simulink model "satellite"  (R2025b)
settings: Solver=ode4  StartTime=0.0  StopTime=100  FixedStep=0.001  RelTol=1e-3
values from neighbouring files (symbols this model uses):
  A_mw = [ ... (first row only)    [init_params.m]
  A_w = [ ... (first row only)    [init_params.m]
  angle0 = eAR'    [init_params.m]
  area_d = 4    [init_params.m]
  area_s = 2    [init_params.m]
  B_mw = [ ... (first row only)    [init_params.m]
  C_bus = 0.001    [init_params.m]
  C_mw = [ ... (first row only)    [init_params.m]
  Cd = 2.2    [init_params.m]
  cos_g_max = cos(gamma_max)    [init_params.m]
  Cr = 1.2    [init_params.m]
  D_max = 0.95    [init_params.m]
  D_min = V_bus_ref / V_oc    (= 0.677637947725)    [init_params.m]
  Delta_D = 0.001    [init_params.m]
  dP_th = 0.05    [init_params.m]
  eta = 0.7    [init_params.m]
  eta_buck = 0.9    [init_params.m]
  eta_chg = 0.95    [init_params.m]
  f = 2.2e9    (= 2200000000)    [init_params.m]
  Gr_dB = 20    [init_params.m]
  Gt_dB = 3    [init_params.m]
  H = 50e3    (= 50000)    [init_params.m]
  h_ref = 400e3    (= 400000)    [init_params.m]
  hat_s = [1;0;0]    [init_params.m]
  I_chg_max = 8    [init_params.m]
  I_dis_max = 10    [init_params.m]
  I_sc = 10.38    [init_params.m]
  Iw = 0.02    [init_params.m]
  J2 = 1.08262668e-3    (= 0.00108262668)    [init_params.m]
  Jx = 10    [init_params.m]
  Jy = 12    [init_params.m]
  Jz = 8    [init_params.m]
  K_w = -A_w' * inv(A_w * A_w')    [init_params.m]
  Kd = [ ... (first row only)    [init_params.m]
  Kp = [ ... (first row only)    [init_params.m]
  m = 500    [init_params.m]
  mu = 3.986004418e14    (= 398600441800000)    [init_params.m]
  n_solar = [1;0;0]    [init_params.m]
  omegaE = 7.2921159e-5    (= 7.2921159e-05)    [init_params.m]
  P0 = 4.56e-6    (= 4.56e-06)    [init_params.m]
  P_adcs = 20    [init_params.m]
  P_base = 50    [init_params.m]
  P_cc = 220/V_bus_ref    (= 7.85714285714)    [init_params.m]
  P_comm = 40    [init_params.m]
  P_trickle = 14/V_bus_ref    (= 0.5)    [init_params.m]
  Pt_dBW = 10    [init_params.m]
  Q = 20    [init_params.m]
  Q0 = [0.6;0.8;0;0]    [init_params.m]
  Rb = 0.2    [init_params.m]
  Re = 6378137    [init_params.m]
  rho_ref = 3e-12    [init_params.m]
  SOC0 = 0.6    [init_params.m]
  SOC1 = 0.2    [init_params.m]
  SOC2 = 0.8    [init_params.m]
  SOC_low_adcs = 0.1    [init_params.m]
  SOC_low_comm = 0.2    [init_params.m]
  sta_vec = Re * [ ... (first row only)    [init_params.m]
  T_max = 0.05    [init_params.m]
  V_bus_ref = 28    [init_params.m]
  V_max = 33    [init_params.m]
  V_min = 24    [init_params.m]
  V_oc = 41.32    [init_params.m]
  vx0 = 0    [init_params.m]
  vy0 = 7546    [init_params.m]
  vz0 = 0    [init_params.m]
  w0 = [0;0;0]    [init_params.m]
  x0 = 7e6    (= 7000000)    [init_params.m]
  y0 = 0    [init_params.m]
  z0 = 0    [init_params.m]
libraries: matrix_library x8
settings Model: PauseTimes=900  Creator=NUAA  LastModifiedBy=NUAA

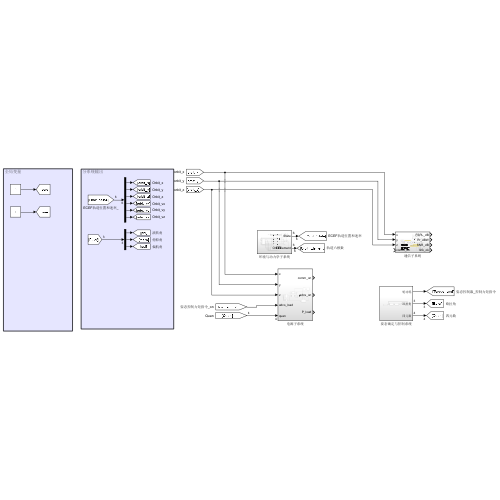
[thumbnail: Simulink's stored preview of the top-level diagram]
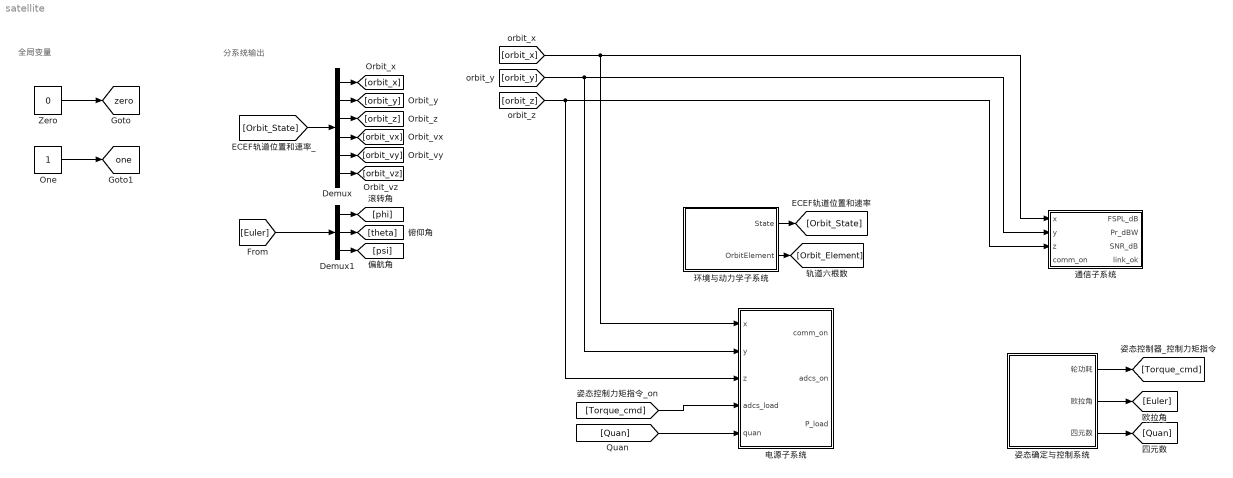
== system satellite ==
  note: 全局变量
  note: 分系统输出
  Demux : Demux  Outputs=6
  Demux1 : Demux  Outputs=3
  One : Constant  OutDataTypeStr=Inherit: Inherit via back propagation
  Zero : Constant  Value=0  OutDataTypeStr=Inherit: Inherit via back propagation
  姿态确定与控制系统 : Subsystem
  环境与动力学子系统 : Subsystem
  电源子系统 : Subsystem
  通信子系统 : Subsystem
  tag scope: one=global, zero=global
  wires:
  环境与动力学子系统/1(State) -> [Orbit_State]
  Demux/1 -> [orbit_x]
  Demux/2 -> [orbit_y]
  Demux/3 -> [orbit_z]
  Demux/4 -> [orbit_vx]
  Demux/5 -> [orbit_vy]
  Demux/6 -> [orbit_vz]
  环境与动力学子系统/2(OrbitElement) -> [Orbit_Element]
  [Orbit_State] -> Demux/1
  [orbit_x] -> 通信子系统/1(x), 电源子系统/1(x)
  [orbit_y] -> 电源子系统/2(y), 通信子系统/2(y)
  姿态确定与控制系统/1(轮功耗) -> [Torque_cmd]
  [Torque_cmd] -> 电源子系统/4(adcs_load)
  [orbit_z] -> 电源子系统/3(z), 通信子系统/3(z)
  姿态确定与控制系统/2(欧拉角) -> [Euler]
  [Euler] -> Demux1/1
  Demux1/1 -> [phi]
  Demux1/2 -> [theta]
  Demux1/3 -> [psi]
  姿态确定与控制系统/3(四元数) -> [Quan]
  [Quan] -> 电源子系统/5(quan)
  Zero/1 -> [zero]
  One/1 -> [one]

== system satellite/姿态确定与控制系统 ==
  Constant1 : Constant  Value=[0;1;0;0]
  三轴PD控制器 : Subsystem
  三轴姿态动力学子系统 : Subsystem
  金字塔反作用轮组件 : Subsystem
  轮功耗 : Outport
  欧拉角 : Outport  Port=2
  四元数 : Outport  Port=3
  wires:
  三轴PD控制器/1(指令力矩) -> 金字塔反作用轮组件/1(指令力矩)
  金字塔反作用轮组件/1(实际力矩) -> 三轴姿态动力学子系统/1(实际力矩)
  金字塔反作用轮组件/3(轮功耗) -> 轮功耗/1
  Constant1/1 -> 三轴PD控制器/3(期望四元数)
  三轴姿态动力学子系统/1(四元数) -> 四元数/1, 三轴PD控制器/1(实际四元数)
  三轴姿态动力学子系统/2(角速率) -> 三轴PD控制器/2(实际角速率)
  三轴姿态动力学子系统/3(欧拉数) -> 欧拉角/1

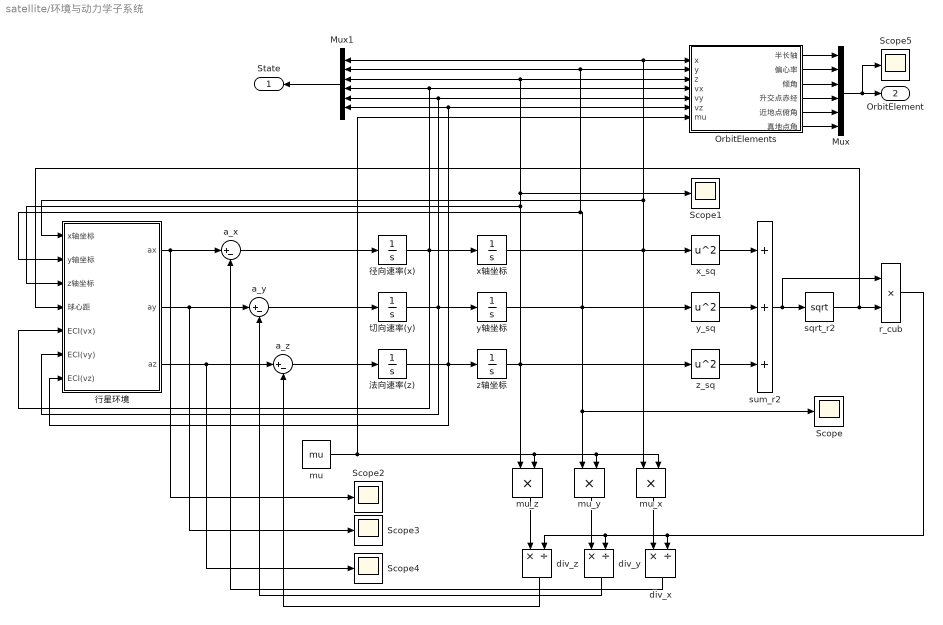
== system satellite/环境与动力学子系统 ==
  Mux : Mux  Inputs=6
  Mux1 : Mux  Inputs=6
  OrbitElements : Subsystem
  Scope{,1..5} (6 alike) : Scope
      Scope settings: ActiveDisplayYMinimum=-187189.8553941616  ActiveDisplayYMaximum=1.6847086985474546E+6
      Scope1 settings: ActiveDisplayYMinimum=-1  ActiveDisplayYMaximum=1
      Scope2 settings: ActiveDisplayYMinimum=-0.013724281044010926  ActiveDisplayYMaximum=0.013844629394884804  DataLoggingVariableName=ScopeData2
      Scope3 settings: ActiveDisplayYMinimum=-0.013784437757224171  ActiveDisplayYMaximum=0.013784949077631064  DataLoggingVariableName=ScopeData3
      Scope4 settings: ActiveDisplayYMinimum=-1  ActiveDisplayYMaximum=1  DataLoggingVariableName=ScopeData4
      Scope5 settings: ActiveDisplayYMinimum=6.9998946797292521E+6  ActiveDisplayYMaximum=6.999959222130728E+6  DataLoggingVariableName=ScopeData5
  a_x : Sum  Inputs=|+-
  a_y : Sum  Inputs=|+-
  a_z : Sum  Inputs=|+-
  div_x : Product  Inputs=*/
  div_y : Product  Inputs=*/
  div_z : Product  Inputs=*/
  mu : Constant  Value=mu
  mu_x : Product
  mu_y : Product
  mu_z : Product
  r_cub : Product
  sqrt_r2 : Sqrt
  sum_r2 : Sum  Inputs=+++
  x_sq : Math  Operator=square
  x轴坐标 : Integrator  InitialCondition=x0
  y_sq : Math  Operator=square
  y轴坐标 : Integrator  InitialCondition=y0
  z_sq : Math  Operator=square
  z轴坐标 : Integrator  InitialCondition=z0
  切向速率(y) : Integrator  InitialCondition=vy0
  径向速率(x) : Integrator  InitialCondition=vx0
  法向速率(z) : Integrator  InitialCondition=vz0
  行星环境 : Subsystem
  State : Outport
  OrbitElement : Outport  Port=2
  wires:
  径向速率(x)/1 -> OrbitElements/4(vx), Mux1/4, 行星环境/5(ECI(vx)), x轴坐标/1
  切向速率(y)/1 -> OrbitElements/5(vy), Mux1/5, 行星环境/6(ECI(vy)), y轴坐标/1
  法向速率(z)/1 -> OrbitElements/6(vz), Mux1/6, 行星环境/7(ECI(vz)), z轴坐标/1
  y轴坐标/1 -> y_sq/1, OrbitElements/2(y), Mux1/2, 行星环境/2(y轴坐标), mu_y/1, Scope/1
  x_sq/1 -> sum_r2/1
  y_sq/1 -> sum_r2/2
  z_sq/1 -> sum_r2/3
  sum_r2/1 -> sqrt_r2/1, r_cub/1
  sqrt_r2/1 -> 行星环境/4(球心距), r_cub/2
  mu_z/1 -> div_z/1
  mu_y/1 -> div_y/1
  mu_x/1 -> div_x/1
  r_cub/1 -> div_x/2, div_y/2, div_z/2
  div_z/1 -> a_z/2
  a_z/1 -> 法向速率(z)/1
  a_y/1 -> 切向速率(y)/1
  div_y/1 -> a_y/2
  div_x/1 -> a_x/2
  x轴坐标/1 -> x_sq/1, mu_x/1, OrbitElements/1(x), Mux1/1, 行星环境/1(x轴坐标)
  z轴坐标/1 -> z_sq/1, Scope1/1, OrbitElements/3(z), Mux1/3, 行星环境/3(z轴坐标), mu_z/1
  行星环境/1(ax) -> a_x/1, Scope2/1
  行星环境/2(ay) -> a_y/1, Scope3/1
  行星环境/3(az) -> a_z/1, Scope4/1
  a_x/1 -> 径向速率(x)/1
  OrbitElements/1(半长轴) -> Mux/1
  OrbitElements/2(偏心率) -> Mux/2
  OrbitElements/3(倾角) -> Mux/3
  OrbitElements/4(升交点赤经) -> Mux/4
  OrbitElements/5(近地点俯角) -> Mux/5
  OrbitElements/6(真地点角) -> Mux/6
  Mux/1 -> OrbitElement/1, Scope5/1
  mu/1 -> OrbitElements/7(mu), mu_x/2, mu_y/2, mu_z/2
  Mux1/1 -> State/1

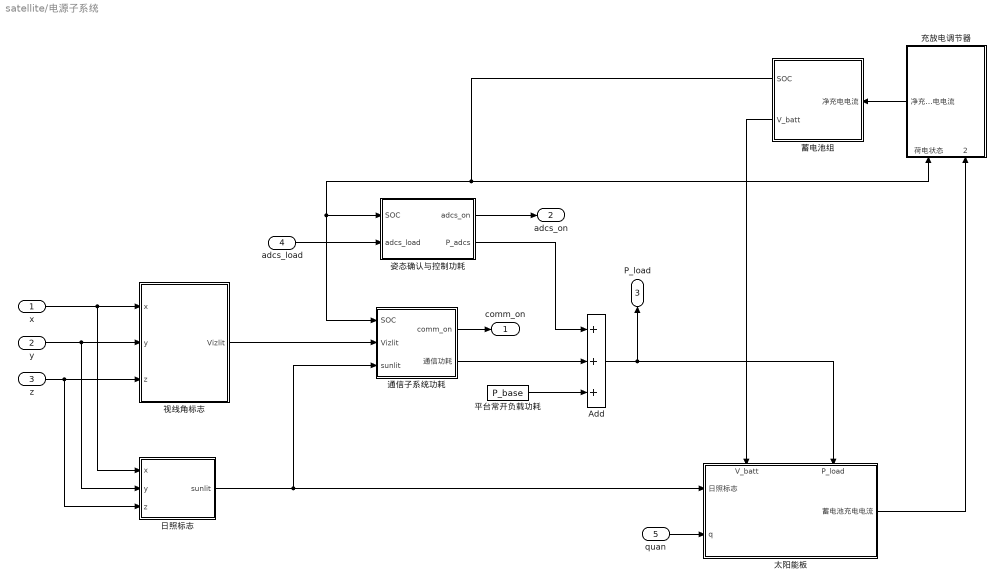
== system satellite/电源子系统 ==
  x : Inport
  y : Inport  Port=2
  z : Inport  Port=3
  adcs_load : Inport  Port=4
  quan : Inport  Port=5
  Add : Sum  Inputs=+++
  充放电调节器 : Subsystem
      settings: PortSchema="{\"entries\":[{\"content\":{\"sides\":[{\"content\":{\"connectorIds\":[\"In1\",\"In2\"]},\"type\":\"ConnectorPlacement.EquallySpacedRectSide\",\"uuid\":\"1ee7afef-72a2-44d7-b1fe-f775c1bd2fb5\"},{\"content\":{\"side\":\"RIGHT\"},\"type\":\"ConnectorPlacement.EquallySpacedRectSide\",\"uuid\":\"a705df99-5add-4aef-8a58-2d39c82bf6d7\"},{\"content\":{\"connectorIds\":[\"Out1\"],\"side\":\"TOP\"},\"type\":\"ConnectorPlacement.EquallySpacedRectSide\",\"uuid\":\"759de5c5-d633-4c5d-bf74-673abcd24ad6\"}]},\"type\":\"ConnectorPlacement.EquallySpacedConnector\",\"uuid\":\"7ef34a9a-0568-4899-98ec-73e8b4fd5653\"}],\"packageUris\":[\"http://schema.mathworks.com/mf0/Connector/R2020b\"],\"version\":\"1.0\"}"
  太阳能板 : Subsystem
      settings: PortSchema="{\"entries\":[{\"content\":{\"sides\":[{\"content\":{\"connectorIds\":[\"In1\",\"In2\"]},\"type\":\"ConnectorPlacement.EquallySpacedRectSide\",\"uuid\":\"5bc779c2-c30f-4cae-b4e1-f2edac4125bf\"},{\"content\":{\"connectorIds\":[\"Out1\"],\"side\":\"RIGHT\"},\"type\":\"ConnectorPlacement.EquallySpacedRectSide\",\"uuid\":\"cdc54232-7dcb-45bf-9570-abbf77ba5ff8\"},{\"content\":{\"connectorIds\":[\"In3\",\"In4\"],\"side\":\"TOP\"},\"type\":\"ConnectorPlacement.EquallySpacedRectSide\",\"uuid\":\"7ae4bd94-3445-4ae2-aeac-bc49ea099582\"}]},\"type\":\"ConnectorPlacement.EquallySpacedConnector\",\"uuid\":\"4dec81bf-3de5-48e4-88d8-77ff2b0205f0\"}],\"packageUris\":[\"http://schema.mathworks.com/mf0/Connector/R2020b\"],\"version\":\"1.0\"}"
  姿态确认与控制功耗 : Subsystem
  平台常开负载功耗 : Constant  Value=P_base
  日照标志 : Subsystem
  蓄电池组 : Subsystem
      settings: PortSchema="{\"entries\":[{\"content\":{\"sides\":[{\"content\":{},\"type\":\"ConnectorPlacement.EquallySpacedRectSide\",\"uuid\":\"7e7ce6a8-f422-4b44-b417-981bf143e596\"},{\"content\":{\"side\":\"RIGHT\"},\"type\":\"ConnectorPlacement.EquallySpacedRectSide\",\"uuid\":\"32e18879-bd9f-43be-9339-7cab6907b877\"},{\"content\":{\"connectorIds\":[\"Out1\",\"Out2\"],\"side\":\"TOP\"},\"type\":\"ConnectorPlacement.EquallySpacedRectSide\",\"uuid\":\"64b37c81-2d28-4322-9005-45a88751c011\"},{\"content\":{\"connectorIds\":[\"In1\"],\"side\":\"BOTTOM\"},\"type\":\"ConnectorPlacement.EquallySpacedRectSide\",\"uuid\":\"597055be-0b91-4221-a6e9-97960dc29d81\"}]},\"type\":\"ConnectorPlacement.EquallySpacedConnector\",\"uuid\":\"41982541-c784-41b5-be8a-a88d5d627e5c\"}],\"packageUris\":[\"http://schema.mathworks.com/mf0/Connector/R2020b\"],\"version\":\"1.0\"}"
  视线角标志 : Subsystem
  通信子系统功耗 : Subsystem
  comm_on : Outport
  adcs_on : Outport  Port=2
  P_load : Outport  Port=3
  wires:
  z/1 -> 视线角标志/3(z), 日照标志/3(z)
  x/1 -> 日照标志/1(x), 视线角标志/1(x)
  adcs_load/1 -> 姿态确认与控制功耗/2(adcs_load)
  y/1 -> 视线角标志/2(y), 日照标志/2(y)
  蓄电池组/1(SOC) -> 通信子系统功耗/1(SOC), 姿态确认与控制功耗/1(SOC), 充放电调节器/1(荷电状态)
  视线角标志/1(Vizlit) -> 通信子系统功耗/2(Vizlit)
  日照标志/1(sunlit) -> 通信子系统功耗/3(sunlit), 太阳能板/1(日照标志)
  quan/1 -> 太阳能板/2(q)
  充放电调节器/1(净充电电流) -> 蓄电池组/1(净充电电流)
  姿态确认与控制功耗/1(adcs_on) -> adcs_on/1
  通信子系统功耗/1(comm_on) -> comm_on/1
  太阳能板/1(蓄电池充电电流) -> 充放电调节器/2(蓄电池充电电流)
  姿态确认与控制功耗/2(P_adcs) -> Add/1
  通信子系统功耗/2(通信功耗) -> Add/2
  平台常开负载功耗/1 -> Add/3
  Add/1 -> P_load/1, 太阳能板/4(P_load)
  蓄电池组/2(V_batt) -> 太阳能板/3(V_batt)

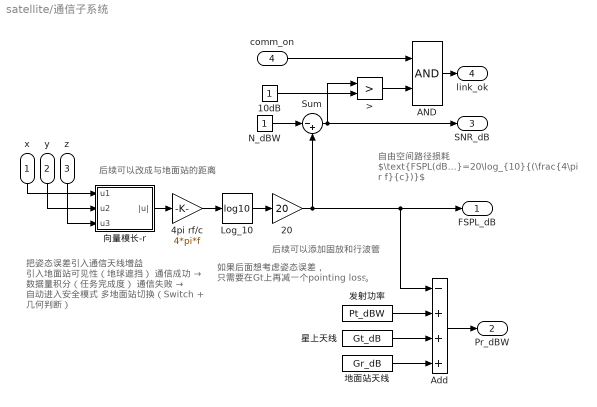
== system satellite/通信子系统 ==
  note: 把姿态误差引入通信天线增益
      | 引入地面站可见性（地球遮挡）
      | 通信成功 → 数据量积分（任务完成度）
      | 通信失败 → 自动进入安全模式
      | 多地面站切换（Switch + 几何判断）
  note: 如果后面想考虑姿态误差，
      | 只需要在Gt上再减一个pointing loss。
  note: 自由空间路径损耗
      | $\text{FSPL(dB)}=20\log_{10}{(\frac{4\pi r f}{c})}$
  note: 后续可以改成与地面站的距离
  note: 后续可以添加固放和行波管
  x : Inport
  y : Inport  Port=2
  z : Inport  Port=3
  comm_on : Inport  Port=4
  10dB : Constant
  20 : Gain  Gain=20
  4pi rf/c : Gain  Gain=4*pi*f
  > : RelationalOperator  Operator=>  OutDataTypeStr=boolean  RndMeth=Simplest  InputSameDT=off
  AND : Logic  AllPortsSameDT=off  OutDataTypeStr=boolean
  Add : Sum  Inputs=-+++
  Log_10 : Math  Operator=log10
  N_dBW : Constant
  Sum : Sum  Inputs=|-+
  发射功率 : Constant  Value=Pt_dBW
  向量模长-r : Subsystem
  地面站天线 : Constant  Value=Gr_dB
  星上天线 : Constant  Value=Gt_dB
  FSPL_dB : Outport
  Pr_dBW : Outport  Port=2
  SNR_dB : Outport  Port=3
  link_ok : Outport  Port=4
  wires:
  x/1 -> 向量模长-r/1(u1)
  y/1 -> 向量模长-r/2(u2)
  z/1 -> 向量模长-r/3(u3)
  向量模长-r/1(|u|) -> 4pi rf/c/1
  4pi rf/c/1 -> Log_10/1
  Log_10/1 -> 20/1
  20/1 -> FSPL_dB/1, Add/1, Sum/2
  发射功率/1 -> Add/2
  星上天线/1 -> Add/3
  地面站天线/1 -> Add/4
  Add/1 -> Pr_dBW/1
  Sum/1 -> SNR_dB/1, >/1
  N_dBW/1 -> Sum/1
  10dB/1 -> >/2
  comm_on/1 -> AND/1
  AND/1 -> link_ok/1
  >/1 -> AND/2

== system satellite/姿态确定与控制系统/三轴PD控制器 ==
  实际四元数 : Inport
  实际角速率 : Inport  Port=2
  期望四元数 : Inport  Port=3
  Demux : Demux
  Mux : Mux  Inputs=3
  Product : Product
  Relay(q0) : Relay  OnOutputValue=-1  OffOutputValue=1
  Sum1 : Sum  Inputs=|+-
  sign(q0) : Signum
  向量逆-qd^-1 : Subsystem
  四元数乘法 : Subsystem
  姿态控制器-微分 : Gain  Gain=Kd
  姿态控制器-比例 : Gain  Gain=Kp
  指令力矩 : Outport
  wires:
  Product/1 -> 姿态控制器-比例/1
  姿态控制器-比例/1 -> Sum1/1
  姿态控制器-微分/1 -> Sum1/2
  Sum1/1 -> 指令力矩/1
  向量逆-qd^-1/1(u^-1) -> 四元数乘法/1(期望逆)
  期望四元数/1 -> 向量逆-qd^-1/1(u)
  实际四元数/1 -> 四元数乘法/2(实际)
  四元数乘法/1(四元数旋转偏差) -> Demux/1
  Demux/1 -> Relay(q0)/1
  Demux/2 -> Mux/1
  Demux/3 -> Mux/2
  Demux/4 -> Mux/3
  Mux/1 -> Product/2
  Relay(q0)/1 -> Product/1
  实际角速率/1 -> 姿态控制器-微分/1

== system satellite/姿态确定与控制系统/三轴姿态动力学子系统 ==
  note: 后续要考虑轨道角速度和部件角动量
  note: 后续可以换成陀螺仪和星敏
  实际力矩 : Inport
  Int_p : Integrator  InitialCondition=w0(1)
  Int_q : Integrator  InitialCondition=w0(1)
  Int_r : Integrator  InitialCondition=w0(3)
  J_x : Gain  Gain=1/Jx
  J_y : Gain  Gain=1/Jy
  J_z : Gain  Gain=1/Jz
  Scope : Scope
      settings: ActiveDisplayYMinimum=-0.23182380450040302  ActiveDisplayYMaximum=2.0864142405036277  DataLoggingVariableName=ScopeData11
  Scope1 : Scope
      settings: ActiveDisplayYMinimum=-0.138741589708908  ActiveDisplayYMaximum=1.1265268433009898  DataLoggingVariableName=ScopeData6
  T(x,y,z) : Demux  Outputs=3
  四元数传播 : Subsystem
  欧拉数传播 : Subsystem
  航天器角速率 : Mux  Inputs=3
  四元数 : Outport
  角速率 : Outport  Port=2
  欧拉数 : Outport  Port=3
  wires:
  实际力矩/1 -> T(x,y,z)/1
  T(x,y,z)/1 -> J_x/1
  T(x,y,z)/2 -> J_y/1
  T(x,y,z)/3 -> J_z/1
  J_x/1 -> Int_p/1
  J_y/1 -> Int_q/1
  J_z/1 -> Int_r/1
  Int_p/1 -> 航天器角速率/1
  Int_q/1 -> 航天器角速率/2
  Int_r/1 -> 航天器角速率/3
  航天器角速率/1 -> 四元数传播/1(机体系角速度分量), 角速率/1, 欧拉数传播/1(机体系角速度分量)
  四元数传播/1(四元数) -> Scope1/1, 四元数/1
  欧拉数传播/1(三轴欧拉角) -> 欧拉数/1, Scope/1

== system satellite/姿态确定与控制系统/金字塔反作用轮组件 ==
  note: 后续可以换成双闭环速度伺服系统
  指令力矩 : Inport
  1/eta : Gain  Gain=1/eta
  Abs : Abs  SaturateOnIntegerOverflow=off
  Product : Product
  State-Space : StateSpace  A=A_mw  B=B_mw  C=C_mw  D=zeros(4,4)  InitialCondition=0
  Sum of Elements : Sum  Inputs=+
  分配矩阵 : Gain  Gain=K_w  Multiplication=Matrix(K*u)
  力矩限幅 : Saturate  UpperLimit=T_max  LowerLimit=-T_max
  安装矩阵 : Gain  Gain=-A_w  Multiplication=Matrix(K*u)
  轮转动惯量 : Gain  Gain=-1/Iw
  轮速积分 : Integrator
  实际力矩 : Outport
  轮速 : Outport  Port=2
  轮功耗 : Outport  Port=3
  wires:
  轮转动惯量/1 -> 轮速积分/1
  State-Space/1 -> 力矩限幅/1
  轮速积分/1 -> Product/2, 轮速/1
  Product/1 -> Abs/1
  力矩限幅/1 -> 安装矩阵/1, Product/1, 轮转动惯量/1
  安装矩阵/1 -> 实际力矩/1
  分配矩阵/1 -> State-Space/1
  指令力矩/1 -> 分配矩阵/1
  Abs/1 -> Sum of Elements/1
  Sum of Elements/1 -> 1/eta/1
  1/eta/1 -> 轮功耗/1

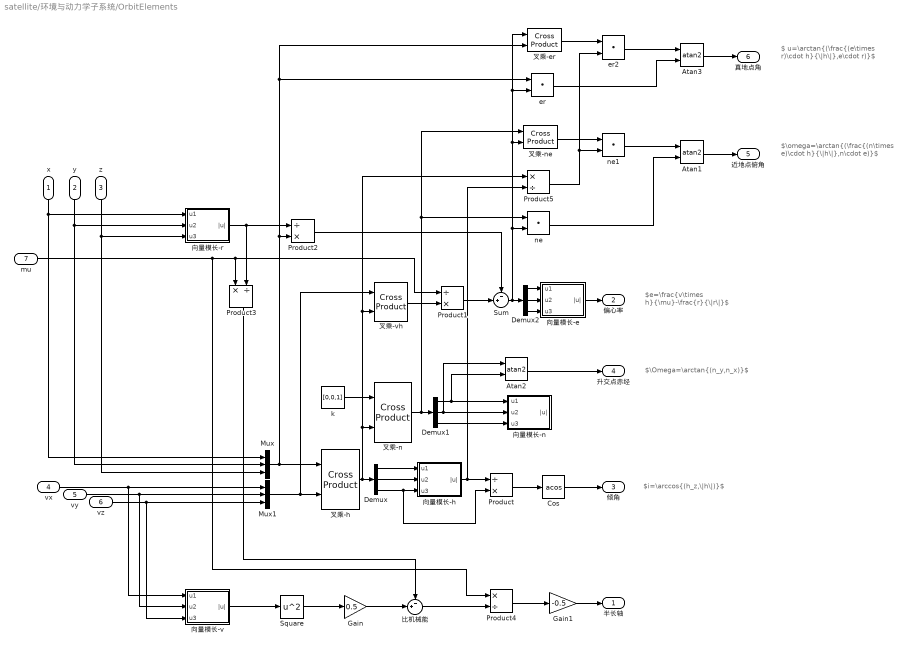
== system satellite/环境与动力学子系统/OrbitElements ==
  note: $i=\arccos{(h_z,\|h\|)}$
  note: $\Omega=\arctan{(n_y,n_x)}$
  note: $e=\frac{v\times h}{\mu}-\frac{r}{\|r\|}$
  note: $\nu=\arctan{(\frac{(e\times r)\cdot h}{\|h\|},e\cdot r)}$
  note: $\omega=\arctan{(\frac{(n\times e)\cdot h}{\|h\|},n\cdot e)}$
  x : Inport
  y : Inport  Port=2
  z : Inport  Port=3
  vx : Inport  Port=4
  vy : Inport  Port=5
  vz : Inport  Port=6
  mu : Inport  Port=7
  Atan1 : Trigonometry  Operator=atan2
  Atan2 : Trigonometry  Operator=atan2
  Atan3 : Trigonometry  Operator=atan2
  Cos : Trigonometry  Operator=acos
  Demux : Demux  Outputs=3
  Demux1 : Demux  Outputs=3
  Demux2 : Demux  Outputs=3
  Gain : Gain  Gain=0.5
  Gain1 : Gain  Gain=-0.5
  Mux : Mux  Inputs=3
  Mux1 : Mux  Inputs=3
  Product : Product  Inputs=/*
  Product1 : Product  Inputs=/*
  Product2 : Product  Inputs=/*
  Product3 : Product  Inputs=*/
  Product4 : Product  Inputs=*/
  Product5 : Product  Inputs=*/
  Square : Math  Operator=square
  Sum : Sum  Inputs=-+|
  er : DotProduct  OutDataTypeStr=Inherit: Inherit via internal rule
  er2 : DotProduct  OutDataTypeStr=Inherit: Inherit via internal rule
  k : Constant  Value=[0,0,1]
  ne : DotProduct  OutDataTypeStr=Inherit: Inherit via internal rule
  ne1 : DotProduct  OutDataTypeStr=Inherit: Inherit via internal rule
  叉乘-er : matrix_library/Cross Product
  叉乘-h : matrix_library/Cross Product
  叉乘-n : matrix_library/Cross Product
  叉乘-ne : matrix_library/Cross Product
  叉乘-vh : matrix_library/Cross Product
  向量模长-e : Subsystem
  向量模长-h : Subsystem
  向量模长-n : Subsystem
  向量模长-r : Subsystem
  向量模长-v : Subsystem
  比机械能 : Sum  Inputs=-+|
  半长轴 : Outport
  偏心率 : Outport  Port=2
  倾角 : Outport  Port=3
  升交点赤经 : Outport  Port=4
  近地点俯角 : Outport  Port=5
  真地点角 : Outport  Port=6
  wires:
  Product/1 -> Cos/1
  向量模长-h/1(|u|) -> Product/1, Product5/2
  Demux/2 -> 向量模长-h/2(u2)
  z/1 -> Mux/3, 向量模长-r/3(u3)
  vx/1 -> Mux1/1, 向量模长-v/1(u1)
  y/1 -> Mux/2, 向量模长-r/2(u2)
  vy/1 -> 向量模长-v/2(u2), Mux1/2
  x/1 -> Mux/1, 向量模长-r/1(u1)
  vz/1 -> Mux1/3, 向量模长-v/3(u3)
  Mux/1 -> er/1, 叉乘-er/2, Product2/2, 叉乘-h/1
  Demux/1 -> 向量模长-h/1(u1)
  Mux1/1 -> 叉乘-h/2, 叉乘-vh/1
  Demux/3 -> Product/2, 向量模长-h/3(u3)
  Cos/1 -> 倾角/1
  叉乘-h/1 -> Product5/1, 叉乘-vh/2, 叉乘-n/2, Demux/1
  叉乘-n/1 -> ne/1, 叉乘-ne/1, Demux1/1
  k/1 -> 叉乘-n/1
  Demux1/1 -> Atan2/2, 向量模长-n/1(u1)
  Demux1/2 -> Atan2/1, 向量模长-n/2(u2)
  Demux1/3 -> 向量模长-n/3(u3)
  Atan2/1 -> 升交点赤经/1
  叉乘-vh/1 -> Product1/2
  mu/1 -> Product4/1, Product3/1, Product1/1
  向量模长-r/1(|u|) -> Product3/2, Product2/1
  Product1/1 -> Sum/2
  Product2/1 -> Sum/1
  Demux2/1 -> 向量模长-e/1(u1)
  Demux2/2 -> 向量模长-e/2(u2)
  Demux2/3 -> 向量模长-e/3(u3)
  向量模长-e/1(|u|) -> 偏心率/1
  向量模长-v/1(|u|) -> Square/1
  Square/1 -> Gain/1
  Gain/1 -> 比机械能/2
  Product3/1 -> 比机械能/1
  Product4/1 -> Gain1/1
  比机械能/1 -> Product4/2
  Gain1/1 -> 半长轴/1
  叉乘-ne/1 -> ne1/1
  ne1/1 -> Atan1/1
  ne/1 -> Atan1/2
  Atan1/1 -> 近地点俯角/1
  Sum/1 -> ne/2, er/2, 叉乘-er/1, 叉乘-ne/2, Demux2/1
  叉乘-er/1 -> er2/1
  er2/1 -> Atan3/1
  er/1 -> Atan3/2
  Atan3/1 -> 真地点角/1
  Product5/1 -> er2/2, ne1/2

== system satellite/环境与动力学子系统/行星环境 ==
  x轴坐标 : Inport
  y轴坐标 : Inport  Port=2
  z轴坐标 : Inport  Port=3
  球心距 : Inport  Port=4
  ECI(vx) : Inport  Port=5
  ECI(vy) : Inport  Port=6
  ECI(vz) : Inport  Port=7
  Add : Sum  Inputs=+++
  Add1 : Sum  Inputs=+++
  Add2 : Sum  Inputs=+++
  J2摄动 : Subsystem
  Mux : Mux  Inputs=3
  大气阻力摄动 : Subsystem
  太阳光压摄动 : Subsystem
  ax : Outport
  ay : Outport  Port=2
  az : Outport  Port=3
  wires:
  x轴坐标/1 -> J2摄动/1(x轴坐标), 大气阻力摄动/1(x轴坐标), Mux/1
  y轴坐标/1 -> J2摄动/2(y轴坐标), 大气阻力摄动/2(y轴坐标), Mux/2
  z轴坐标/1 -> J2摄动/3(z轴坐标), Mux/3
  球心距/1 -> 太阳光压摄动/1(球心距), 大气阻力摄动/3(球心距), J2摄动/4(球心距)
  ECI(vx)/1 -> 大气阻力摄动/4(径向速率(x))
  ECI(vy)/1 -> 大气阻力摄动/5(切向速率(y))
  ECI(vz)/1 -> 大气阻力摄动/6(法向速率(z))
  J2摄动/1(J2x) -> Add/1
  大气阻力摄动/1(Dx) -> Add/2
  Add/1 -> ax/1
  J2摄动/2(J2y) -> Add1/1
  大气阻力摄动/2(Dy) -> Add1/2
  Add1/1 -> ay/1
  J2摄动/3(J2z) -> Add2/1
  大气阻力摄动/3(Dz) -> Add2/2
  Add2/1 -> az/1
  Mux/1 -> 太阳光压摄动/2(三轴坐标)
  太阳光压摄动/1(srp_x) -> Add/3
  太阳光压摄动/2(srp_y) -> Add1/3
  太阳光压摄动/3(srp_z) -> Add2/3

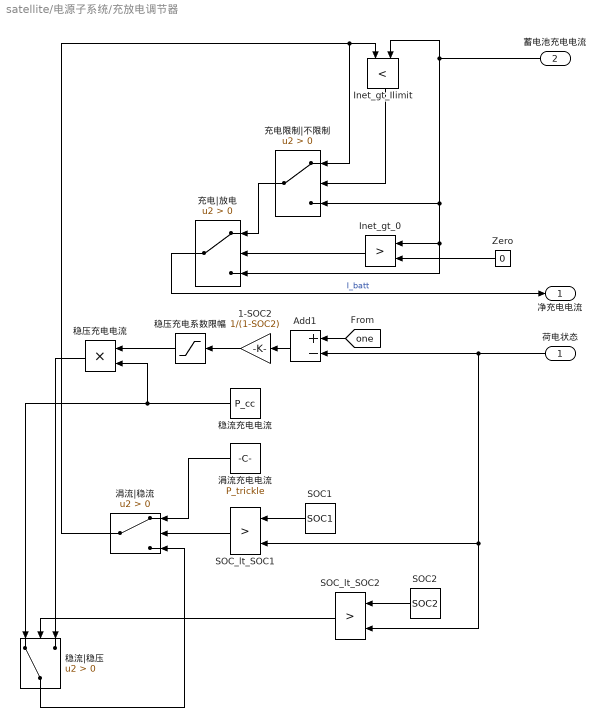
== system satellite/电源子系统/充放电调节器 ==
  荷电状态 : Inport
  蓄电池充电电流 : Inport  Port=2
  1-SOC2 : Gain  Gain=1/(1-SOC2)
  Add1 : Sum  Inputs=+-
  Inet_gt_0 : RelationalOperator  Operator=>  OutDataTypeStr=boolean  RndMeth=Simplest  InputSameDT=off
  Inet_gt_Ilimit : RelationalOperator  Operator=<  OutDataTypeStr=boolean  RndMeth=Simplest  InputSameDT=off
  SOC1 : Constant  Value=SOC1
  SOC2 : Constant  Value=SOC2
  SOC_lt_SOC1 : RelationalOperator  Operator=>  OutDataTypeStr=boolean  RndMeth=Simplest  InputSameDT=off
  SOC_lt_SOC2 : RelationalOperator  Operator=>  OutDataTypeStr=boolean  RndMeth=Simplest  InputSameDT=off
  Zero : Constant  Value=0  OutDataTypeStr=Inherit: Inherit via back propagation
  充电|放电 : Switch  Criteria=u2 > Threshold  SaturateOnIntegerOverflow=off  InputSameDT=off
  充电限制|不限制 : Switch  Criteria=u2 > Threshold  SaturateOnIntegerOverflow=off  InputSameDT=off
  涓流|稳流 : Switch  Criteria=u2 > Threshold  SaturateOnIntegerOverflow=off  InputSameDT=off
  涓流充电电流 : Constant  Value=P_trickle
  稳压充电电流 : Product
  稳压充电系数限幅 : Saturate  UpperLimit=1  LowerLimit=0
  稳流|稳压 : Switch  Criteria=u2 > Threshold  SaturateOnIntegerOverflow=off  InputSameDT=off
  稳流充电电流 : Constant  Value=P_cc
  净充电电流 : Outport
  wires:
  [one] -> Add1/1
  蓄电池充电电流/1 -> Inet_gt_Ilimit/2, 充电|放电/3, Inet_gt_0/1, 充电限制|不限制/3
  SOC_lt_SOC2/1 -> 稳流|稳压/2
  稳压充电电流/1 -> 稳流|稳压/3
  Inet_gt_Ilimit/1 -> 充电限制|不限制/2
  荷电状态/1 -> SOC_lt_SOC2/2, SOC_lt_SOC1/2, Add1/2
  稳流充电电流/1 -> 稳压充电电流/2, 稳流|稳压/1
  1-SOC2/1 -> 稳压充电系数限幅/1
  涓流|稳流/1 -> 充电限制|不限制/1, Inet_gt_Ilimit/1
  SOC_lt_SOC1/1 -> 涓流|稳流/2
  充电|放电/1 -> 净充电电流/1  "I_batt"
  Inet_gt_0/1 -> 充电|放电/2
  充电限制|不限制/1 -> 充电|放电/1
  Add1/1 -> 1-SOC2/1
  SOC1/1 -> SOC_lt_SOC1/1
  SOC2/1 -> SOC_lt_SOC2/1
  稳压充电系数限幅/1 -> 稳压充电电流/1
  涓流充电电流/1 -> 涓流|稳流/1
  稳流|稳压/1 -> 涓流|稳流/3
  Zero/1 -> Inet_gt_0/2

== system satellite/电源子系统/太阳能板 ==
  note: 最简单的光生电流，后续可改为
      | $I_{pannel}=I_{ph}-I_0\left( e^{\frac{V_{pannel}+IR_s}{nV_t}} -1\right)-\frac{V_{pannel}+IR_s}{R_{sh}}$
  日照标志 : Inport
  q : Inport  Port=2
  V_batt : Inport  Port=3
  P_load : Inport  Port=4
  Add2 : Sum  Inputs=+--
  Gain : Gain  Gain=1/C_bus
  Gain1 : Gain  Gain=1/Rb
  Integrator : Integrator  InitialCondition=V_bus_ref
  Product3 : Product  Inputs=*/
  Saturation : Saturate  UpperLimit=I_chg_max  LowerLimit=-I_dis_max
  Sum : Sum  Inputs=|-+
  太阳板 : Subsystem
  母线电压 : Saturate  UpperLimit=inf  LowerLimit=0
  蓄电池充电电流 : Outport
  wires:
  P_load/1 -> Product3/1
  太阳板/1(太阳板输出电流) -> Add2/1
  Product3/1 -> Add2/3  "I_load"
  Gain1/1 -> Saturation/1
  Saturation/1 -> 蓄电池充电电流/1, Add2/2  "蓄电池充电电流"
  Add2/1 -> Gain/1
  Gain/1 -> Integrator/1
  Integrator/1 -> 母线电压/1
  母线电压/1 -> Sum/2, 太阳板/3(母线电压), Product3/2  "V_bus"
  V_batt/1 -> Sum/1
  Sum/1 -> Gain1/1
  q/1 -> 太阳板/1(q)
  日照标志/1 -> 太阳板/2(日照标志)

== system satellite/电源子系统/姿态确认与控制功耗 ==
  SOC : Inport
  adcs_load : Inport  Port=2
  0.01 : Constant  Value=0.01
  AND : Logic  AllPortsSameDT=off  OutDataTypeStr=boolean
  Add2 : Sum
  SOC_adcs_1/0 : Relay  OnSwitchValue=SOC_low_adcs + 0.02  OffSwitchValue=SOC_low_adcs
  Switch : Switch  Criteria=u2 > Threshold  SaturateOnIntegerOverflow=off  InputSameDT=off
  T_gt_001 : RelationalOperator  Operator=<=  OutDataTypeStr=boolean  RndMeth=Simplest  InputSameDT=off
  姿态开时负载功耗 : Constant  Value=P_adcs
  adcs_on : Outport
  P_adcs : Outport  Port=2
  wires:
  Switch/1 -> P_adcs/1
  adcs_load/1 -> Add2/1, T_gt_001/2
  AND/1 -> adcs_on/1, Switch/2
  Add2/1 -> Switch/1
  0.01/1 -> T_gt_001/1
  姿态开时负载功耗/1 -> Add2/2
  [zero] -> Switch/3
  T_gt_001/1 -> AND/1
  SOC_adcs_1/0/1 -> AND/2
  SOC/1 -> SOC_adcs_1/0/1

== system satellite/电源子系统/日照标志 ==
  x : Inport
  y : Inport  Port=2
  z : Inport  Port=3
  Add1 : Sum
  Sqrt : Sqrt
  Square : Math  Operator=square
  Square1 : Math  Operator=square
  Zero : Constant  Value=0  OutDataTypeStr=Inherit: Inherit via back propagation
  abs_y_lt_Re : RelationalOperator  Operator=<  OutDataTypeStr=boolean  RndMeth=Simplest  InputSameDT=off
  and_sclipse : Logic  AllPortsSameDT=off  OutDataTypeStr=boolean
  not_sunlit : Logic  Operator=NOT  AllPortsSameDT=off  OutDataTypeStr=boolean
  x_lt_0 : RelationalOperator  Operator=<  OutDataTypeStr=boolean  RndMeth=Simplest  InputSameDT=off
  地球半径 : Constant  Value=Re
  sunlit : Outport
  wires:
  and_sclipse/1 -> not_sunlit/1
  abs_y_lt_Re/1 -> and_sclipse/2
  地球半径/1 -> abs_y_lt_Re/2
  Square1/1 -> Add1/2
  Square/1 -> Add1/1
  Sqrt/1 -> abs_y_lt_Re/1
  Add1/1 -> Sqrt/1
  x_lt_0/1 -> and_sclipse/1
  x/1 -> x_lt_0/1
  z/1 -> Square1/1
  y/1 -> Square/1
  not_sunlit/1 -> sunlit/1
  Zero/1 -> x_lt_0/2

== system satellite/电源子系统/蓄电池组 ==
  净充电电流 : Inport
  Add3 : Sum
  Constant : Constant  Value=V_max-V_min
  Constant1 : Constant  Value=V_min
  DIV_SOC : Gain  Gain=1/(Q*3600)
  Product : Product
  Relay : Relay
  SOC_delay : Memory  InitialCondition=SOC0
  Scope2 : Scope
      settings: ActiveDisplayYMinimum=0.61855578548532641  ActiveDisplayYMaximum=0.62097219625968636  DataLoggingVariableName=ScopeData9
  Switch : Switch  Criteria=u2 > Threshold  SaturateOnIntegerOverflow=off  InputSameDT=off
  int_SOC : Integrator  InitialCondition=SOC0  LimitOutput=on  UpperSaturationLimit=1  LowerSaturationLimit=0
  充电效率 : Gain  Gain=eta_chg
  放电效率 : Gain  Gain=1/eta_chg
  SOC : Outport
  V_batt : Outport  Port=2
  wires:
  净充电电流/1 -> 放电效率/1, 充电效率/1, Relay/1
  Switch/1 -> DIV_SOC/1
  充电效率/1 -> Switch/1
  Relay/1 -> Switch/2
  放电效率/1 -> Switch/3
  SOC_delay/1 -> Product/1, Scope2/1, SOC/1
  DIV_SOC/1 -> int_SOC/1
  int_SOC/1 -> SOC_delay/1
  Product/1 -> Add3/1
  Constant/1 -> Product/2
  Constant1/1 -> Add3/2
  Add3/1 -> V_batt/1

== system satellite/电源子系统/视线角标志 ==
  x : Inport
  y : Inport  Port=2
  z : Inport  Port=3
  Mux : Mux  Inputs=3
  余弦夹角 : Subsystem
  地面站向量 : Constant  Value=sta_vec
  小于最大视角 : RelationalOperator  OutDataTypeStr=boolean  RndMeth=Simplest  InputSameDT=off
  最大视线角 : Constant  Value=cos_g_max
  Vizlit : Outport
  wires:
  地面站向量/1 -> 余弦夹角/1(u1)
  Mux/1 -> 余弦夹角/2(u2)
  小于最大视角/1 -> Vizlit/1
  最大视线角/1 -> 小于最大视角/2
  余弦夹角/1(cos(γ)) -> 小于最大视角/1
  x/1 -> Mux/1
  y/1 -> Mux/2
  z/1 -> Mux/3

== system satellite/电源子系统/通信子系统功耗 ==
  SOC : Inport
  Vizlit : Inport  Port=2
  sunlit : Inport  Port=3
  AND1 : Logic  Inputs=3  AllPortsSameDT=off  OutDataTypeStr=boolean
  SOC_comm_1/0 : Relay  OnSwitchValue=SOC_low_comm + 0.02  OffSwitchValue=SOC_low_comm
  Switch : Switch  Criteria=u2 > Threshold  SaturateOnIntegerOverflow=off  InputSameDT=off
  通信开时负载功耗 : Constant  Value=P_comm
  comm_on : Outport
  通信功耗 : Outport  Port=2
  wires:
  AND1/1 -> Switch/2, comm_on/1
  sunlit/1 -> AND1/3
  通信开时负载功耗/1 -> Switch/1
  SOC_comm_1/0/1 -> AND1/1
  Switch/1 -> 通信功耗/1
  SOC/1 -> SOC_comm_1/0/1
  Vizlit/1 -> AND1/2
  [zero] -> Switch/3

== system satellite/通信子系统/向量模长-r ==
  u1 : Inport
  u2 : Inport  Port=2
  u3 : Inport  Port=3
  Add : Sum  Inputs=+++
  Sqrt : Sqrt
  Square : Math  Operator=square
  Square1 : Math  Operator=square
  Square2 : Math  Operator=square
  |u| : Outport
  wires:
  u1/1 -> Square/1
  u2/1 -> Square1/1
  u3/1 -> Square2/1
  Square/1 -> Add/1
  Square1/1 -> Add/2
  Square2/1 -> Add/3
  Add/1 -> Sqrt/1
  Sqrt/1 -> |u|/1

== system satellite/姿态确定与控制系统/三轴PD控制器/向量逆-qd^-1 ==
  u : Inport
  -qd1 : Gain  Gain=-1
  -qd2 : Gain  Gain=-1
  -qd3 : Gain  Gain=-1
  Demux : Demux
  Mux : Mux
  u^-1 : Outport
  wires:
  u/1 -> Demux/1
  Mux/1 -> u^-1/1
  Demux/1 -> Mux/1
  Demux/2 -> -qd1/1
  -qd1/1 -> Mux/2
  Demux/3 -> -qd2/1
  -qd2/1 -> Mux/3
  Demux/4 -> -qd3/1
  -qd3/1 -> Mux/4

== system satellite/姿态确定与控制系统/三轴PD控制器/四元数乘法 ==
  期望逆 : Inport
  实际 : Inport  Port=2
  Add : Sum  Inputs=3
  Cross Product : matrix_library/Cross Product
  Demux : Demux
  Demux1 : Demux
  Dot Product : DotProduct  OutDataTypeStr=Inherit: Inherit via internal rule
  Mux : Mux  Inputs=2
  Mux1 : Mux  Inputs=3
  Mux2 : Mux  Inputs=3
  Product : Product
  Product1 : Product
  Product2 : Product
  Sum : Sum  Inputs=|+-
  四元数旋转偏差 : Outport
  wires:
  期望逆/1 -> Demux/1
  实际/1 -> Demux1/1
  Mux/1 -> 四元数旋转偏差/1
  Product/1 -> Sum/1
  Demux/1 -> Product1/1, Product/1
  Mux1/1 -> Dot Product/1, Cross Product/1, Product2/2
  Demux1/1 -> Product2/1, Product/2
  Mux2/1 -> Cross Product/2, Dot Product/2, Product1/2
  Sum/1 -> Mux/1
  Dot Product/1 -> Sum/2
  Product2/1 -> Add/2
  Product1/1 -> Add/1
  Cross Product/1 -> Add/3
  Add/1 -> Mux/2
  Demux/2 -> Mux1/1
  Demux/3 -> Mux1/2
  Demux/4 -> Mux1/3
  Demux1/2 -> Mux2/1
  Demux1/3 -> Mux2/2
  Demux1/4 -> Mux2/3

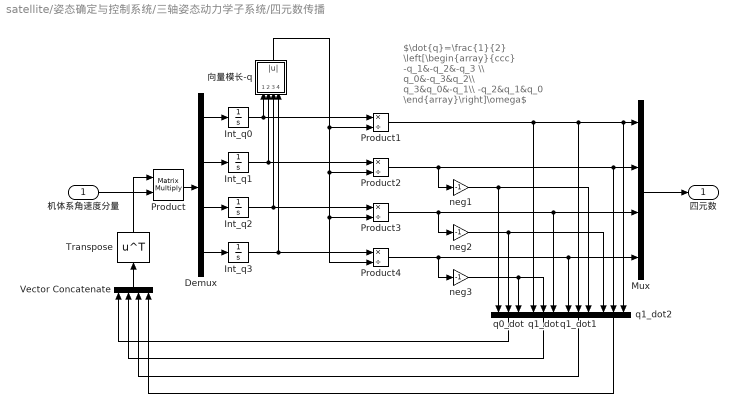
== system satellite/姿态确定与控制系统/三轴姿态动力学子系统/四元数传播 ==
  note: $\dot{q}=\frac{1}{2} \left[\begin{array}{ccc} -q_1&-q_2&-q_3 \\ q_0&-q_3&q_2\\ q_3&q_0&-q_1\\ -q_2&q_1&q_0 \end{array}\right]\omega$
  机体系角速度分量 : Inport
  Demux : Demux
  Int_q0 : Integrator  InitialCondition=Q0(1)
  Int_q1 : Integrator  InitialCondition=Q0(2)
  Int_q2 : Integrator  InitialCondition=Q0(3)
  Int_q3 : Integrator  InitialCondition=Q0(4)
  Mux : Mux
  Product : Product  Multiplication=Matrix(*)
  Product{1..4} (4 alike) : Product  Inputs=*/
  Transpose : Math  Operator=transpose
  Vector Concatenate : Concatenate  NumInputs=4  Mode=Multidimensional array  ConcatenateDimension=2
  neg1 : Gain  Gain=-1
  neg2 : Gain  Gain=-1
  neg3 : Gain  Gain=-1
  q0_dot : Mux  Inputs=3
  q1_dot : Mux  Inputs=3
  q1_dot1 : Mux  Inputs=3
  q1_dot2 : Mux  Inputs=3
  向量模长-q : Subsystem
  四元数 : Outport
  wires:
  Product/1 -> Demux/1
  neg1/1 -> q0_dot/1, q1_dot1/3
  q1_dot/1 -> Vector Concatenate/2
  neg3/1 -> q1_dot/2, q0_dot/3
  Product4/1 -> neg3/1, Mux/4, q1_dot1/1
  Product1/1 -> q1_dot/1, q1_dot1/2, Mux/1, q1_dot2/3
  q1_dot1/1 -> Vector Concatenate/3
  Demux/2 -> Int_q1/1
  Product2/1 -> neg1/1, q1_dot2/2, Mux/2
  Demux/3 -> Int_q2/1
  neg2/1 -> q1_dot2/1, q0_dot/2
  q1_dot2/1 -> Vector Concatenate/4
  Product3/1 -> neg2/1, Mux/3, q1_dot/3
  Mux/1 -> 四元数/1
  q0_dot/1 -> Vector Concatenate/1
  Vector Concatenate/1 -> Transpose/1
  Demux/1 -> Int_q0/1
  Demux/4 -> Int_q3/1
  机体系角速度分量/1 -> Product/2
  Transpose/1 -> Product/1
  Int_q0/1 -> Product1/1, 向量模长-q/1(u0)
  Int_q1/1 -> Product2/1, 向量模长-q/2(u1)
  Int_q2/1 -> Product3/1, 向量模长-q/3(u2)
  Int_q3/1 -> Product4/1, 向量模长-q/4(u3)
  向量模长-q/1(|u|) -> Product2/2, Product3/2, Product4/2, Product1/2

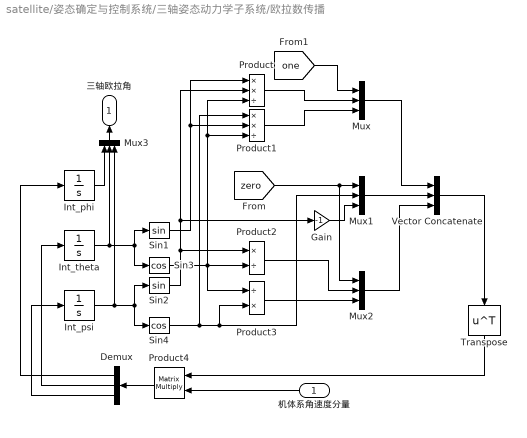
== system satellite/姿态确定与控制系统/三轴姿态动力学子系统/欧拉数传播 ==
  机体系角速度分量 : Inport
  Demux : Demux  Outputs=3
  Gain : Gain  Gain=-1
  Int_phi : Integrator  InitialCondition=angle0(1)
  Int_psi : Integrator  InitialCondition=angle0(3)
  Int_theta : Integrator  InitialCondition=angle0(2)
  Mux{,1..3} (4 alike) : Mux  Inputs=3
  Product : Product  Inputs=**/
  Product1 : Product  Inputs=**/
  Product2 : Product  Inputs=*/
  Product3 : Product  Inputs=/*
  Product4 : Product  Multiplication=Matrix(*)
  Sin1 : Trigonometry
  Sin2 : Trigonometry
  Sin3 : Trigonometry  Operator=cos
  Sin4 : Trigonometry  Operator=cos
  Transpose : Math  Operator=transpose
  Vector Concatenate : Concatenate  NumInputs=3  Mode=Multidimensional array  ConcatenateDimension=2
  三轴欧拉角 : Outport
  wires:
  Mux2/1 -> Vector Concatenate/3
  Gain/1 -> Mux1/3
  Demux/1 -> Int_phi/1
  [one] -> Mux/1
  Demux/3 -> Int_psi/1
  Demux/2 -> Int_theta/1
  Int_psi/1 -> Mux3/3, Sin4/1, Sin2/1
  Sin1/1 -> Product/1, Product1/2
  Product1/1 -> Mux/3
  Sin4/1 -> Product3/2, Mux1/2, Product1/1
  Int_theta/1 -> Sin3/1, Sin1/1, Mux3/2
  Sin2/1 -> Product/2, Gain/1, Product2/1
  Mux/1 -> Vector Concatenate/1
  Sin3/1 -> Product/3, Product1/3, Product2/2, Product3/1
  Mux1/1 -> Vector Concatenate/2
  Product3/1 -> Mux2/3
  Vector Concatenate/1 -> Transpose/1
  Product2/1 -> Mux2/2
  [zero] -> Mux2/1, Mux1/1
  机体系角速度分量/1 -> Product4/2
  Product/1 -> Mux/2
  Product4/1 -> Demux/1
  Int_phi/1 -> Mux3/1
  Mux3/1 -> 三轴欧拉角/1
  Transpose/1 -> Product4/1

== system satellite/环境与动力学子系统/OrbitElements/向量模长-e ==
  u1 : Inport
  u2 : Inport  Port=2
  u3 : Inport  Port=3
  Add : Sum  Inputs=+++
  Sqrt : Sqrt
  Square : Math  Operator=square
  Square1 : Math  Operator=square
  Square2 : Math  Operator=square
  |u| : Outport
  wires:
  u1/1 -> Square/1
  u2/1 -> Square1/1
  u3/1 -> Square2/1
  Square/1 -> Add/1
  Square1/1 -> Add/2
  Square2/1 -> Add/3
  Add/1 -> Sqrt/1
  Sqrt/1 -> |u|/1

== system satellite/环境与动力学子系统/OrbitElements/向量模长-h ==
  u1 : Inport
  u2 : Inport  Port=2
  u3 : Inport  Port=3
  Add : Sum  Inputs=+++
  Sqrt : Sqrt
  Square : Math  Operator=square
  Square1 : Math  Operator=square
  Square2 : Math  Operator=square
  |u| : Outport
  wires:
  Sqrt/1 -> |u|/1
  Add/1 -> Sqrt/1
  Square2/1 -> Add/3
  Square1/1 -> Add/2
  Square/1 -> Add/1
  u3/1 -> Square2/1
  u2/1 -> Square1/1
  u1/1 -> Square/1

== system satellite/环境与动力学子系统/OrbitElements/向量模长-n ==
  u1 : Inport
  u2 : Inport  Port=2
  u3 : Inport  Port=3
  Add : Sum  Inputs=+++
  Sqrt : Sqrt
  Square : Math  Operator=square
  Square1 : Math  Operator=square
  Square2 : Math  Operator=square
  |u| : Outport
  wires:
  u1/1 -> Square/1
  u2/1 -> Square1/1
  u3/1 -> Square2/1
  Square/1 -> Add/1
  Square1/1 -> Add/2
  Square2/1 -> Add/3
  Add/1 -> Sqrt/1
  Sqrt/1 -> |u|/1

== system satellite/环境与动力学子系统/OrbitElements/向量模长-r ==
  u1 : Inport
  u2 : Inport  Port=2
  u3 : Inport  Port=3
  Add : Sum  Inputs=+++
  Sqrt : Sqrt
  Square : Math  Operator=square
  Square1 : Math  Operator=square
  Square2 : Math  Operator=square
  |u| : Outport
  wires:
  u1/1 -> Square/1
  u2/1 -> Square1/1
  u3/1 -> Square2/1
  Square/1 -> Add/1
  Square1/1 -> Add/2
  Square2/1 -> Add/3
  Add/1 -> Sqrt/1
  Sqrt/1 -> |u|/1

== system satellite/环境与动力学子系统/OrbitElements/向量模长-v ==
  u1 : Inport
  u2 : Inport  Port=2
  u3 : Inport  Port=3
  Add : Sum  Inputs=+++
  Sqrt : Sqrt
  Square : Math  Operator=square
  Square1 : Math  Operator=square
  Square2 : Math  Operator=square
  |u| : Outport
  wires:
  Sqrt/1 -> |u|/1
  Add/1 -> Sqrt/1
  Square2/1 -> Add/3
  Square1/1 -> Add/2
  Square/1 -> Add/1
  u3/1 -> Square2/1
  u2/1 -> Square1/1
  u1/1 -> Square/1

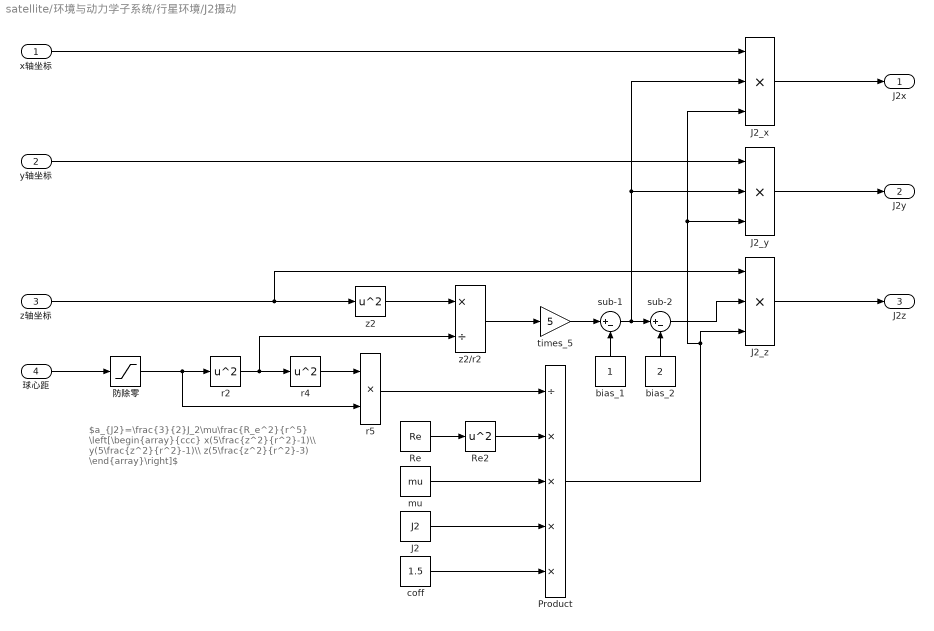
== system satellite/环境与动力学子系统/行星环境/J2摄动 ==
  note: $a_{J2}=\frac{3}{2}J_2\mu\frac{R_e^2}{r^5} \left[\begin{array}{ccc} x(5\frac{z^2}{r^2}-1)\\ y(5\frac{z^2}{r^2}-1)\\ z(5\frac{z^2}{r^2}-3) \end{array}\right]$
  x轴坐标 : Inport
  y轴坐标 : Inport  Port=2
  z轴坐标 : Inport  Port=3
  球心距 : Inport  Port=4
  J2 : Constant  Value=J2
  J2_x : Product  Inputs=3
  J2_y : Product  Inputs=3
  J2_z : Product  Inputs=3
  Product : Product  Inputs=/****
  Re : Constant  Value=Re
  Re2 : Math  Operator=square
  bias_1 : Constant
  bias_2 : Constant  Value=2
  coff : Constant  Value=1.5
  mu : Constant  Value=mu
  r2 : Math  Operator=square
  r4 : Math  Operator=square
  r5 : Product
  sub-1 : Sum  Inputs=|+-
  sub-2 : Sum  Inputs=|+-
  times_5 : Gain  Gain=5
  z2 : Math  Operator=square
  z2/r2 : Product  Inputs=*/
  防除零 : Saturate  UpperLimit=inf  LowerLimit=Re+80e3
  J2x : Outport
  J2y : Outport  Port=2
  J2z : Outport  Port=3
  wires:
  Re2/1 -> Product/2
  z2/1 -> z2/r2/1
  x轴坐标/1 -> J2_x/1
  z2/r2/1 -> times_5/1
  sub-1/1 -> J2_y/2, J2_x/2, sub-2/1
  Product/1 -> J2_x/3, J2_y/3, J2_z/3
  coff/1 -> Product/5
  J2_z/1 -> J2z/1
  r4/1 -> r5/1
  z轴坐标/1 -> J2_z/1, z2/1
  r2/1 -> z2/r2/2, r4/1
  球心距/1 -> 防除零/1
  bias_1/1 -> sub-1/2
  mu/1 -> Product/3
  times_5/1 -> sub-1/1
  sub-2/1 -> J2_z/2
  Re/1 -> Re2/1
  y轴坐标/1 -> J2_y/1
  J2/1 -> Product/4
  r5/1 -> Product/1
  bias_2/1 -> sub-2/2
  J2_y/1 -> J2y/1
  J2_x/1 -> J2x/1
  防除零/1 -> r5/2, r2/1

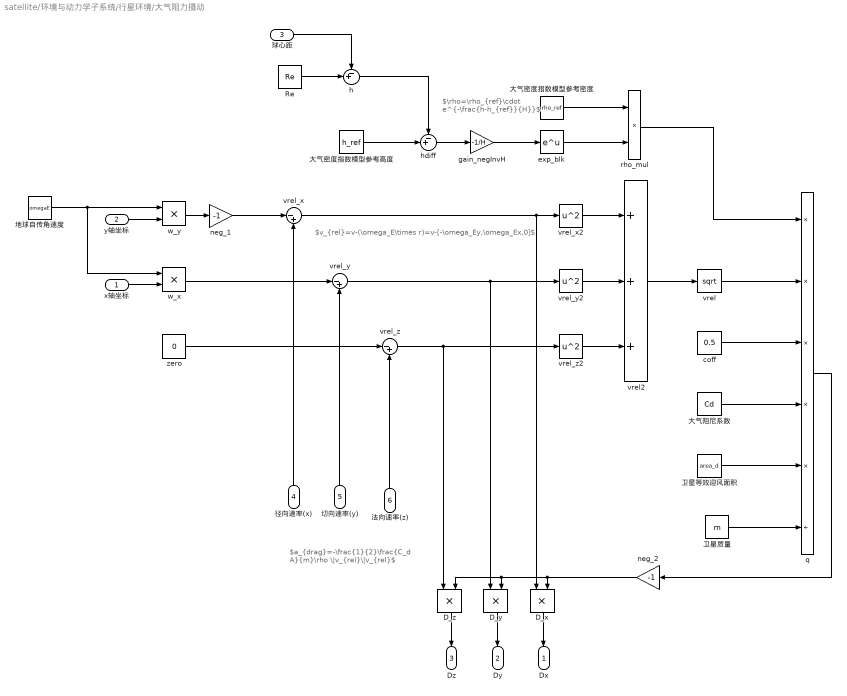
== system satellite/环境与动力学子系统/行星环境/大气阻力摄动 ==
  note: $a_{drag}=-\frac{1}{2}\frac{C_d A}{m}\rho \|v_{rel}\|v_{rel}$
  note: $\rho=\rho_{ref}\cdot e^{-\frac{h-h_{ref}}{H}}$
  note: $v_{rel}=v-(\omega_E\times r)=v-[-\omega_Ey,\omega_Ex,0]$
  x轴坐标 : Inport
  y轴坐标 : Inport  Port=2
  球心距 : Inport  Port=3
  径向速率(x) : Inport  Port=4
  切向速率(y) : Inport  Port=5
  法向速率(z) : Inport  Port=6
  D_x : Product
  D_y : Product
  D_z : Product
  Re : Constant  Value=Re
  coff : Constant  Value=0.5
  exp_blk : Math
  gain_negInvH : Gain  Gain=-1/H
  h : Sum  Inputs=-+|
  hdiff : Sum  Inputs=-+|
  neg_1 : Gain  Gain=-1
  neg_2 : Gain  Gain=-1
  q : Product  Inputs=*****/
  rho_mul : Product
  vrel : Sqrt
  vrel2 : Sum  Inputs=+++
  vrel_x : Sum  Inputs=|-+
  vrel_x2 : Math  Operator=square
  vrel_y : Sum  Inputs=|-+
  vrel_y2 : Math  Operator=square
  vrel_z : Sum  Inputs=|-+
  vrel_z2 : Math  Operator=square
  w_x : Product
  w_y : Product
  zero : Constant  Value=0
  卫星等效迎风面积 : Constant  Value=area_d
  卫星质量 : Constant  Value=m
  地球自传角速度 : Constant  Value=omegaE
  大气密度指数模型参考密度 : Constant  Value=rho_ref
  大气密度指数模型参考高度 : Constant  Value=h_ref
  大气阻尼系数 : Constant  Value=Cd
  Dx : Outport
  Dy : Outport  Port=2
  Dz : Outport  Port=3
  wires:
  法向速率(z)/1 -> vrel_z/2
  切向速率(y)/1 -> vrel_y/2
  w_y/1 -> neg_1/1
  vrel_x/1 -> D_x/1, vrel_x2/1
  q/1 -> neg_2/1
  vrel_z2/1 -> vrel2/3
  vrel_x2/1 -> vrel2/1
  大气密度指数模型参考密度/1 -> rho_mul/1
  vrel2/1 -> vrel/1
  Re/1 -> h/2
  地球自传角速度/1 -> w_x/1, w_y/1
  x轴坐标/1 -> w_x/2
  neg_1/1 -> vrel_x/1
  vrel_y/1 -> D_y/1, vrel_y2/1
  D_z/1 -> Dz/1
  vrel_y2/1 -> vrel2/2
  coff/1 -> q/3
  rho_mul/1 -> q/1
  h/1 -> hdiff/1
  w_x/1 -> vrel_y/1
  卫星质量/1 -> q/6
  卫星等效迎风面积/1 -> q/5
  gain_negInvH/1 -> exp_blk/1
  zero/1 -> vrel_z/1
  径向速率(x)/1 -> vrel_x/2
  vrel_z/1 -> D_z/1, vrel_z2/1
  大气密度指数模型参考高度/1 -> hdiff/2
  hdiff/1 -> gain_negInvH/1
  vrel/1 -> q/2
  大气阻尼系数/1 -> q/4
  exp_blk/1 -> rho_mul/2
  y轴坐标/1 -> w_y/2
  球心距/1 -> h/1
  D_x/1 -> Dx/1
  D_y/1 -> Dy/1
  neg_2/1 -> D_x/2, D_y/2, D_z/2

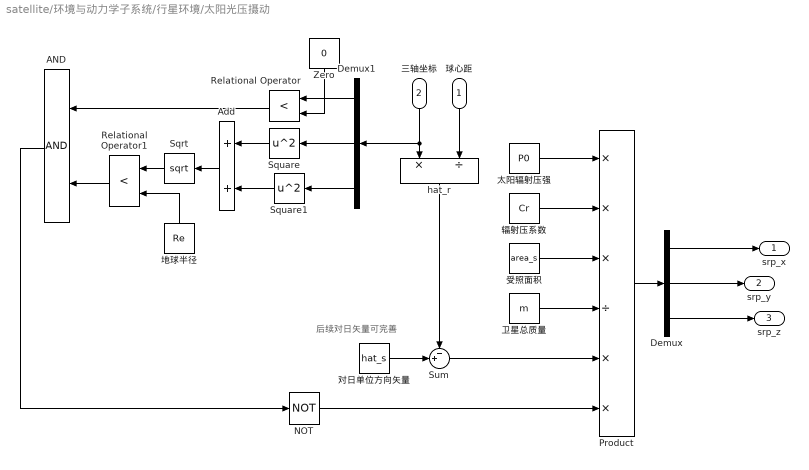
== system satellite/环境与动力学子系统/行星环境/太阳光压摄动 ==
  note: 后续对日矢量可完善
  球心距 : Inport
  三轴坐标 : Inport  Port=2
  AND : Logic  AllPortsSameDT=off  OutDataTypeStr=boolean
  Add : Sum
  Demux : Demux  Outputs=3
  Demux1 : Demux  Outputs=3
  NOT : Logic  Operator=NOT  AllPortsSameDT=off  OutDataTypeStr=boolean
  Product : Product  Inputs=***/**
  Relational Operator : RelationalOperator  Operator=<  OutDataTypeStr=boolean  RndMeth=Simplest  InputSameDT=off
  Relational Operator1 : RelationalOperator  Operator=<  OutDataTypeStr=boolean  RndMeth=Simplest  InputSameDT=off
  Sqrt : Sqrt
  Square : Math  Operator=square
  Square1 : Math  Operator=square
  Sum : Sum  Inputs=-+|
  Zero : Constant  Value=0  OutDataTypeStr=Inherit: Inherit via back propagation
  hat_r : Product  Inputs=*/
  卫星总质量 : Constant  Value=m
  受照面积 : Constant  Value=area_s
  地球半径 : Constant  Value=Re
  太阳辐射压强 : Constant  Value=P0
  对日单位方向矢量 : Constant  Value=hat_s
  辐射压系数 : Constant  Value=Cr
  srp_x : Outport
  srp_y : Outport  Port=2
  srp_z : Outport  Port=3
  wires:
  Sum/1 -> Product/5
  太阳辐射压强/1 -> Product/1
  卫星总质量/1 -> Product/4
  受照面积/1 -> Product/3
  对日单位方向矢量/1 -> Sum/2
  辐射压系数/1 -> Product/2
  hat_r/1 -> Sum/1
  Product/1 -> Demux/1
  球心距/1 -> hat_r/2
  Demux/3 -> srp_z/1
  Demux/2 -> srp_y/1
  三轴坐标/1 -> Demux1/1, hat_r/1
  Demux/1 -> srp_x/1
  Demux1/1 -> Relational Operator/1
  Zero/1 -> Relational Operator/2
  Demux1/2 -> Square/1
  Demux1/3 -> Square1/1
  Square/1 -> Add/1
  Square1/1 -> Add/2
  Add/1 -> Sqrt/1
  Sqrt/1 -> Relational Operator1/1
  地球半径/1 -> Relational Operator1/2
  Relational Operator1/1 -> AND/2
  Relational Operator/1 -> AND/1
  NOT/1 -> Product/6
  AND/1 -> NOT/1

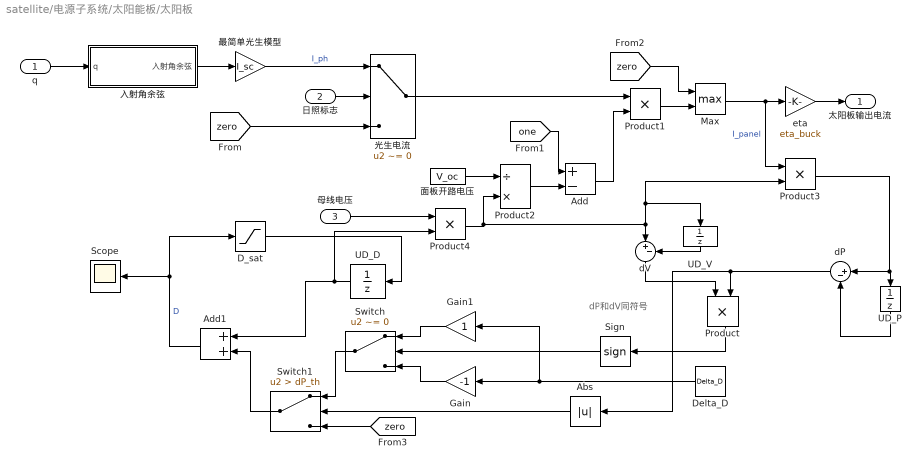
== system satellite/电源子系统/太阳能板/太阳板 ==
  note: dP和dV同符号
  q : Inport
  日照标志 : Inport  Port=2
  母线电压 : Inport  Port=3
  Abs : Abs  SaturateOnIntegerOverflow=off
  Add : Sum  Inputs=+-
  Add1 : Sum
  D_sat : Saturate  UpperLimit=D_max  LowerLimit=D_min
  Delta_D : Constant  Value=Delta_D
  Gain : Gain  Gain=-1
  Gain1 : Gain
  Max : MinMax  Function=max  Inputs=2
  Product : Product
  Product1 : Product
  Product2 : Product  Inputs=/*
  Product3 : Product
  Product4 : Product  Inputs=**
  Scope : Scope
      settings: ActiveDisplayYMinimum=0.25493544986237704  ActiveDisplayYMaximum=0.98361023080225229  DataLoggingVariableName=ScopeData7
  Sign : Signum
  Switch : Switch  Criteria=u2 ~= 0  SaturateOnIntegerOverflow=off  InputSameDT=off
  Switch1 : Switch  Criteria=u2 > Threshold  Threshold=dP_th  SaturateOnIntegerOverflow=off  InputSameDT=off
  UD_D : UnitDelay  SampleTime=-1  HasFrameUpgradeWarning=on
  UD_P : UnitDelay  SampleTime=-1  HasFrameUpgradeWarning=on
  UD_V : UnitDelay  SampleTime=-1  HasFrameUpgradeWarning=on
  dP : Sum  Inputs=|+-
  dV : Sum  Inputs=|+-
  eta : Gain  Gain=eta_buck
  光生电流 : Switch  Criteria=u2 ~= 0  SaturateOnIntegerOverflow=off  InputSameDT=off
  入射角余弦 : Subsystem
  最简单光生模型 : Gain  Gain=I_sc
  面板开路电压 : Constant  Value=V_oc
  太阳板输出电流 : Outport
  wires:
  Product4/1 -> Product2/2, Product3/2, UD_V/1, dV/1
  Add/1 -> Product1/2
  光生电流/1 -> Product1/1
  Product2/1 -> Add/2
  最简单光生模型/1 -> 光生电流/1  "I_ph"
  q/1 -> 入射角余弦/1(q)
  面板开路电压/1 -> Product2/1
  日照标志/1 -> 光生电流/2
  [one] -> Add/1
  [zero] -> Max/1
  入射角余弦/1(入射角余弦) -> 最简单光生模型/1
  [zero] -> 光生电流/3
  Product1/1 -> Max/2
  Max/1 -> Product3/1, eta/1  "I_panel"
  eta/1 -> 太阳板输出电流/1
  dV/1 -> Product/1
  dP/1 -> Abs/1, Product/2
  Product/1 -> Sign/1
  Sign/1 -> Switch/2
  Gain/1 -> Switch/3
  Gain1/1 -> Switch/1
  Delta_D/1 -> Gain1/1, Gain/1
  Product3/1 -> dP/1, UD_P/1
  UD_P/1 -> dP/2
  UD_V/1 -> dV/2
  Switch/1 -> Switch1/1
  UD_D/1 -> Product4/2, Add1/1
  Add1/1 -> Scope/1, D_sat/1  "D"
  母线电压/1 -> Product4/1
  D_sat/1 -> UD_D/1
  Switch1/1 -> Add1/2
  Abs/1 -> Switch1/2
  [zero] -> Switch1/3

== system satellite/电源子系统/视线角标志/余弦夹角 ==
  u1 : Inport
  u2 : Inport  Port=2
  Demux : Demux  Outputs=3
  Demux1 : Demux  Outputs=3
  Dot Product : DotProduct  OutDataTypeStr=Inherit: Inherit via internal rule
  余弦夹角 : Product  Inputs=/*/
  向量模长-r1 : Subsystem
  向量模长-r2 : Subsystem
  cos(γ) : Outport
  wires:
  向量模长-r2/1(|u|) -> 余弦夹角/3
  Demux/3 -> 向量模长-r1/3(u3)
  Demux/2 -> 向量模长-r1/2(u2)
  Dot Product/1 -> 余弦夹角/2
  Demux/1 -> 向量模长-r1/1(u1)
  向量模长-r1/1(|u|) -> 余弦夹角/1
  u2/1 -> Dot Product/2, Demux1/1
  Demux1/1 -> 向量模长-r2/1(u1)
  Demux1/2 -> 向量模长-r2/2(u2)
  Demux1/3 -> 向量模长-r2/3(u3)
  u1/1 -> Dot Product/1, Demux/1
  余弦夹角/1 -> cos(γ)/1

== system satellite/姿态确定与控制系统/三轴姿态动力学子系统/四元数传播/向量模长-q ==
  u0 : Inport
  u1 : Inport  Port=2
  u2 : Inport  Port=3
  u3 : Inport  Port=4
  Add : Sum  Inputs=4
  Sqrt : Sqrt
  Square{,1..3} (4 alike) : Math  Operator=square
  |u| : Outport
  wires:
  u0/1 -> Square/1
  u1/1 -> Square1/1
  u2/1 -> Square2/1
  Square/1 -> Add/1
  Square1/1 -> Add/2
  Square2/1 -> Add/3
  Add/1 -> Sqrt/1
  Sqrt/1 -> |u|/1
  u3/1 -> Square3/1
  Square3/1 -> Add/4

== system satellite/电源子系统/太阳能板/太阳板/入射角余弦 ==
  q : Inport
  Max : MinMax  Function=max  Inputs=2
  余弦夹角1 : Subsystem
  共轭 : Subsystem
  四元数乘法 : Subsystem
  四元数旋转 : Subsystem
  地日矢量 : Constant  Value=[0;hat_s]
  面板法向量 : Constant  Value=n_solar
  入射角余弦 : Outport
  wires:
  四元数旋转/1(Q*) -> 余弦夹角1/2(u2)
  余弦夹角1/1(cos(γ)) -> Max/1
  四元数乘法/1(Q*) -> 四元数旋转/1(Q1)
  q/1 -> 四元数旋转/2(Q2), 共轭/1(q)
  面板法向量/1 -> 余弦夹角1/1(u1)
  共轭/1(q*) -> 四元数乘法/1(Q1)
  地日矢量/1 -> 四元数乘法/2(Q2)
  Max/1 -> 入射角余弦/1
  [zero] -> Max/2

== system satellite/电源子系统/视线角标志/余弦夹角/向量模长-r1 ==
  u1 : Inport
  u2 : Inport  Port=2
  u3 : Inport  Port=3
  Add : Sum  Inputs=+++
  Sqrt : Sqrt
  Square : Math  Operator=square
  Square1 : Math  Operator=square
  Square2 : Math  Operator=square
  |u| : Outport
  wires:
  Sqrt/1 -> |u|/1
  Add/1 -> Sqrt/1
  Square2/1 -> Add/3
  Square1/1 -> Add/2
  Square/1 -> Add/1
  u3/1 -> Square2/1
  u2/1 -> Square1/1
  u1/1 -> Square/1

== system satellite/电源子系统/视线角标志/余弦夹角/向量模长-r2 ==
  u1 : Inport
  u2 : Inport  Port=2
  u3 : Inport  Port=3
  Add : Sum  Inputs=+++
  Sqrt : Sqrt
  Square : Math  Operator=square
  Square1 : Math  Operator=square
  Square2 : Math  Operator=square
  |u| : Outport
  wires:
  u1/1 -> Square/1
  u2/1 -> Square1/1
  u3/1 -> Square2/1
  Square/1 -> Add/1
  Square1/1 -> Add/2
  Square2/1 -> Add/3
  Add/1 -> Sqrt/1
  Sqrt/1 -> |u|/1

== system satellite/电源子系统/太阳能板/太阳板/入射角余弦/余弦夹角1 ==
  u1 : Inport
  u2 : Inport  Port=2
  Demux : Demux  Outputs=3
  Demux1 : Demux  Outputs=3
  Dot Product : DotProduct  OutDataTypeStr=Inherit: Inherit via internal rule
  余弦夹角 : Product  Inputs=/*/
  向量模长-r1 : Subsystem
  向量模长-r2 : Subsystem
  cos(γ) : Outport
  wires:
  向量模长-r2/1(|u|) -> 余弦夹角/3
  Demux/3 -> 向量模长-r1/3(u3)
  Demux/2 -> 向量模长-r1/2(u2)
  Dot Product/1 -> 余弦夹角/2
  Demux/1 -> 向量模长-r1/1(u1)
  向量模长-r1/1(|u|) -> 余弦夹角/1
  u2/1 -> Dot Product/2, Demux1/1
  Demux1/1 -> 向量模长-r2/1(u1)
  Demux1/2 -> 向量模长-r2/2(u2)
  Demux1/3 -> 向量模长-r2/3(u3)
  u1/1 -> Dot Product/1, Demux/1
  余弦夹角/1 -> cos(γ)/1

== system satellite/电源子系统/太阳能板/太阳板/入射角余弦/共轭 ==
  q : Inport
  -qd1 : Gain  Gain=-1
  -qd2 : Gain  Gain=-1
  -qd3 : Gain  Gain=-1
  Demux : Demux
  Mux : Mux
  q* : Outport
  wires:
  q/1 -> Demux/1
  Mux/1 -> q*/1
  Demux/1 -> Mux/1
  Demux/2 -> -qd1/1
  -qd1/1 -> Mux/2
  Demux/3 -> -qd2/1
  -qd2/1 -> Mux/3
  Demux/4 -> -qd3/1
  -qd3/1 -> Mux/4

== system satellite/电源子系统/太阳能板/太阳板/入射角余弦/四元数乘法 ==
  Q1 : Inport
  Q2 : Inport  Port=2
  Add : Sum  Inputs=3
  Cross Product : matrix_library/Cross Product
  Demux : Demux
  Demux1 : Demux
  Dot Product : DotProduct  OutDataTypeStr=Inherit: Inherit via internal rule
  Mux : Mux  Inputs=2
  Mux1 : Mux  Inputs=3
  Mux2 : Mux  Inputs=3
  Product : Product
  Product1 : Product
  Product2 : Product
  Sum : Sum  Inputs=|+-
  Q* : Outport
  wires:
  Q1/1 -> Demux/1
  Q2/1 -> Demux1/1
  Mux/1 -> Q*/1
  Product/1 -> Sum/1
  Demux/1 -> Product1/1, Product/1
  Mux1/1 -> Dot Product/1, Cross Product/1, Product2/2
  Demux1/1 -> Product2/1, Product/2
  Mux2/1 -> Cross Product/2, Dot Product/2, Product1/2
  Sum/1 -> Mux/1
  Dot Product/1 -> Sum/2
  Product2/1 -> Add/2
  Product1/1 -> Add/1
  Cross Product/1 -> Add/3
  Add/1 -> Mux/2
  Demux/2 -> Mux1/1
  Demux/3 -> Mux1/2
  Demux/4 -> Mux1/3
  Demux1/2 -> Mux2/1
  Demux1/3 -> Mux2/2
  Demux1/4 -> Mux2/3

== system satellite/电源子系统/太阳能板/太阳板/入射角余弦/四元数旋转 ==
  Q1 : Inport
  Q2 : Inport  Port=2
  Add : Sum  Inputs=3
  Cross Product : matrix_library/Cross Product
  Demux : Demux
  Demux1 : Demux
  Mux1 : Mux  Inputs=3
  Mux2 : Mux  Inputs=3
  Product1 : Product
  Product2 : Product
  Q* : Outport
  wires:
  Demux1/4 -> Mux2/3
  Demux1/3 -> Mux2/2
  Demux1/2 -> Mux2/1
  Demux/4 -> Mux1/3
  Demux/3 -> Mux1/2
  Demux/2 -> Mux1/1
  Add/1 -> Q*/1
  Cross Product/1 -> Add/3
  Product1/1 -> Add/1
  Product2/1 -> Add/2
  Mux2/1 -> Product1/2, Cross Product/2
  Demux1/1 -> Product2/1
  Mux1/1 -> Product2/2, Cross Product/1
  Demux/1 -> Product1/1
  Q2/1 -> Demux1/1
  Q1/1 -> Demux/1

== system satellite/电源子系统/太阳能板/太阳板/入射角余弦/余弦夹角1/向量模长-r1 ==
  u1 : Inport
  u2 : Inport  Port=2
  u3 : Inport  Port=3
  Add : Sum  Inputs=+++
  Sqrt : Sqrt
  Square : Math  Operator=square
  Square1 : Math  Operator=square
  Square2 : Math  Operator=square
  |u| : Outport
  wires:
  Sqrt/1 -> |u|/1
  Add/1 -> Sqrt/1
  Square2/1 -> Add/3
  Square1/1 -> Add/2
  Square/1 -> Add/1
  u3/1 -> Square2/1
  u2/1 -> Square1/1
  u1/1 -> Square/1

== system satellite/电源子系统/太阳能板/太阳板/入射角余弦/余弦夹角1/向量模长-r2 ==
  u1 : Inport
  u2 : Inport  Port=2
  u3 : Inport  Port=3
  Add : Sum  Inputs=+++
  Sqrt : Sqrt
  Square : Math  Operator=square
  Square1 : Math  Operator=square
  Square2 : Math  Operator=square
  |u| : Outport
  wires:
  u1/1 -> Square/1
  u2/1 -> Square1/1
  u3/1 -> Square2/1
  Square/1 -> Add/1
  Square1/1 -> Add/2
  Square2/1 -> Add/3
  Add/1 -> Sqrt/1
  Sqrt/1 -> |u|/1
